simulink model "L22PendCartsim"  (R2020a)
settings: Solver=FixedStepAuto  StartTime=0.0  StopTime=100  FixedStep=0.001  RelTol=1e-3
InitFcn:
  | L22pendcartparameters;
values from neighbouring files (symbols this model uses):
  A = [0 1 0 0; 0 -d/M m*g/M 0; 0 0 0 1; 0 d/(M*L) -(m+M)*g/(M*L) 0]    [L22pendcartparameters.m]
  B = [0 ; 1/M ; 0 ; -1/(M*L)]    [L22pendcartparameters.m]
  Baug = [B G]    [L22pendcartparameters.m]
  C = [1 0 0 0]    [L22pendcartparameters.m]
  KLQR = lqr(A,B,Q,R)    [L22pendcartparameters.m]
  x0 = [0.5; 0; 0.1; 0]    [L22pendcartparameters.m]
  xhat0 = [0;0;0;0]    [L22pendcartparameters.m]
undefined symbols (not defined in the file or in its folder): LKB
libraries: simulink x2
settings Model: Creator=vcichella  LastModifiedBy=vcichella

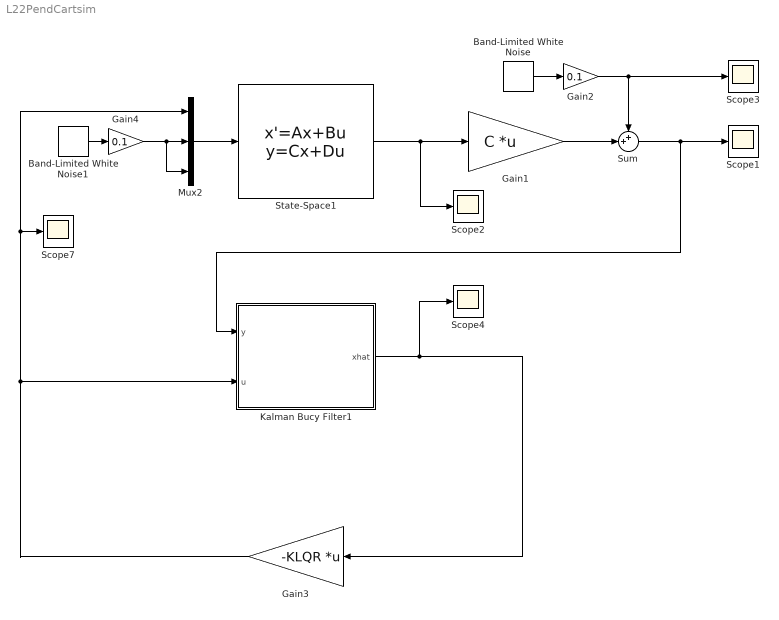
== system L22PendCartsim ==
  Band-Limited White Noise : simulink/Sources/Band-Limited White Noise  Cov=[0.01]  Ts=0.01  seed=[23341]
  Band-Limited White Noise1 : simulink/Sources/Band-Limited White Noise  Cov=[0.0001]  Ts=0.01  seed=[23341]
  Gain1 : Gain  Gain=C  Multiplication=Matrix(K*u)
  Gain2 : Gain  Gain=0.1
  Gain3 : Gain  Gain=-KLQR  Multiplication=Matrix(K*u)
  Gain4 : Gain  Gain=0.1
  Kalman Bucy Filter1 : Subsystem
  Mux2 : Mux  Inputs=3
  Scope{1..4,7} (5 alike) : Scope
  State-Space1 : StateSpace  A=A  B=Baug  C=eye(size(A))  D=zeros(4,3)  InitialCondition=x0
  Sum : Sum  Inputs=++|
  wires:
  State-Space1/1 -> Scope2/1, Gain1/1
  Sum/1 -> Kalman Bucy Filter1/1(y), Scope1/1
  Gain1/1 -> Sum/2
  Band-Limited White Noise/1 -> Gain2/1
  Mux2/1 -> State-Space1/1
  Kalman Bucy Filter1/1(xhat) -> Scope4/1, Gain3/1
  Band-Limited White Noise1/1 -> Gain4/1
  Gain3/1 -> Mux2/1, Scope7/1, Kalman Bucy Filter1/2(u)
  Gain2/1 -> Sum/1, Scope3/1
  Gain4/1 -> Mux2/3, Mux2/2

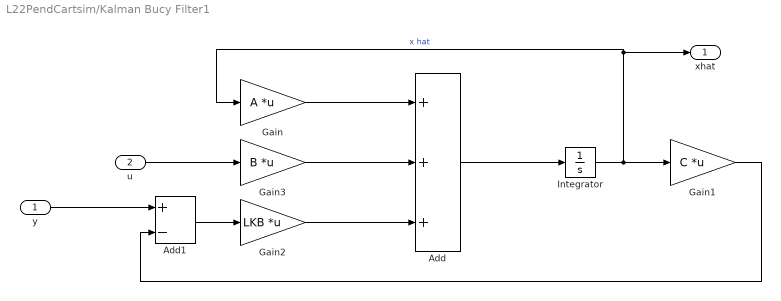
== system L22PendCartsim/Kalman Bucy Filter1 ==
  y : Inport
  u : Inport  Port=2
  Add : Sum  Inputs=+++
  Add1 : Sum  Inputs=+-
  Gain : Gain  Gain=A  Multiplication=Matrix(K*u)
  Gain1 : Gain  Gain=C  Multiplication=Matrix(K*u)
  Gain2 : Gain  Gain=LKB  Multiplication=Matrix(K*u)
  Gain3 : Gain  Gain=B  Multiplication=Matrix(K*u)
  Integrator : Integrator  InitialCondition=xhat0
  xhat : Outport
  wires:
  Integrator/1 -> xhat/1, Gain/1, Gain1/1  "x hat"
  Add/1 -> Integrator/1
  Gain/1 -> Add/1
  Gain1/1 -> Add1/2
  Add1/1 -> Gain2/1
  y/1 -> Add1/1
  Gain2/1 -> Add/3
  u/1 -> Gain3/1
  Gain3/1 -> Add/2
